simulink model "forZeroPurpose"  (R2015a)
settings: Solver=ode45  StartTime=0.0  StopTime=10.0  RelTol=1e-3
values from neighbouring files (symbols this model uses):
  A = [-31.31 0 -2.833e4 2; 0 -10.25 8001 0; 1 -1 0 0; 0 0 0 -100]    [Copy_of_UIE_tracking_main.m]    (also in UIE_main.m = [0 0 1 0; 0 0 0 1; -3 1 -0.4 0.1; 1 -1 0.1 -0.1]; UIE_tracking_main.m = [0 0 1 0; 0 0 0 1; -3 1 -0.4 0.1; 1 -1 0.1 -0.1])
  B = [28.06 0 0 1; 0 28.06 0 1]'    [Copy_of_UIE_tracking_main.m]    (also in UIE_main.m = [0 0; 0 0; 1 0; 0 1]; UIE_tracking_main.m = [0 0; 0 0; 1 0; 0 1])
  C = [1 0 0 0;1 0 30 0]    [Copy_of_UIE_tracking_main.m]    (also in UIE_main.m = [1 0 0 0; 0 1 0 0]; UIE_tracking_main.m = [1 0 0 0; 0 1 0 0])
  Ec = -inv(Rc)*B'*inv(A - B*Kc)'*C'*Qc    [Copy_of_UIE_tracking_main.m]    (also in UIE_main.m; UIE_tracking_main.m)
  Kc = lqr(A + Hc*eye(n), B, C'*Qc*C, Rc)    [Copy_of_UIE_tracking_main.m]    (also in UIE_main.m; UIE_tracking_main.m)
  Tf = 1e-3    (= 0.001)    [Copy_of_UIE_tracking_main.m]    (also in UIE_main.m; UIE_tracking_main.m)
  x_ini = [0 0 0 0]    [Copy_of_UIE_tracking_main.m]    (also in UIE_main.m = [0 1 0 0]; UIE_tracking_main.m)
settings Model: Creator=Elca  LastModifiedBy=Elca

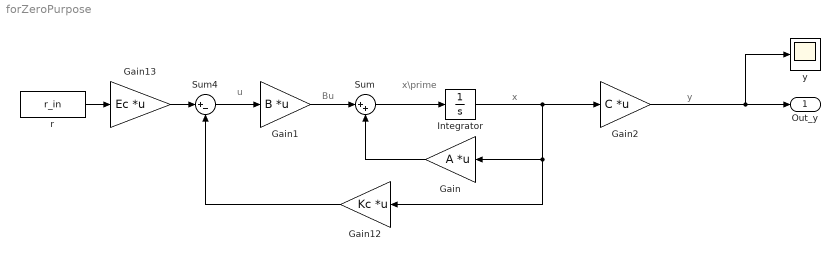
== system forZeroPurpose ==
  note: Bu
  note: x\prime
  note: x
  note: y
  note: u
  Gain : Gain  Gain=A  Multiplication=Matrix(K*u)
  Gain1 : Gain  Gain=B  Multiplication=Matrix(K*u)
  Gain12 : Gain  Gain=Kc  Multiplication=Matrix(K*u)
  Gain13 : Gain  Gain=Ec  Multiplication=Matrix(K*u)
  Gain2 : Gain  Gain=C  Multiplication=Matrix(K*u)
  Integrator : Integrator  InitialCondition=x_ini
  Sum : Sum  Inputs=|++
  Sum4 : Sum  Inputs=|+-
  r : FromWorkspace  VariableName=r_in  SampleTime=Tf
  y : Scope
      settings: TickLabels=on  YMin=0  YMax=550000  SaveName=ScopeData4  ScrollMode=on
  Out_y : Outport
  wires:
  Sum/1 -> Integrator/1
  Integrator/1 -> Gain12/1, Gain/1, Gain2/1
  Gain2/1 -> y/1, Out_y/1
  Gain/1 -> Sum/2
  Gain12/1 -> Sum4/2
  Gain13/1 -> Sum4/1
  r/1 -> Gain13/1
  Sum4/1 -> Gain1/1
  Gain1/1 -> Sum/1
